simulink model "Modelo_SS_Simulink"  (R2025b)
settings: Solver=ode45  StartTime=0.0  StopTime=inf  FixedStep=0.002  RelTol=1e-3
values from neighbouring files (symbols this model uses):
  A = sym(zeros(7,7))    [Analisis_Contr_Obs.m]    (also in Gs_simbolica.m; Modelo_SS.m = zeros(7,7))
  B_SS = [Bc Bd]    [Modelo_SS.m]
  Bc = sym(zeros(7,1))    [Analisis_Contr_Obs.m]    (also in Modelo_SS.m = zeros(7,1))
  C_s = [0 0 0 1 0 0 0]    [Modelo_SS.m]
  C_SS = eye(7)    [Modelo_SS.m]
  D_SS = zeros(7,4)    [Modelo_SS.m]
  Ff_cte = 9    [Modelo_SS.m]
  K_lqr = lqr(A, Bc, Qx, Qu)    [Modelo_SS.m]
  Kf = 26000    [Modelo_SS.m]
  kr = -1 / (C_p * ((A - Bc*K_lqr) \ Bc))    [Modelo_SS.m]
  Kt = 0.6    [Modelo_SS.m]
  rL = 0.115    [Modelo_SS.m]
  Rm = 0.135    [Modelo_SS.m]
  rP = rP_kin    (= 0.00509295817894)    [Modelo_SS.m]
  tau_sensor = 0.001    [Modelo_SS.m]
  Tf_cte = 2    [Modelo_SS.m]
  Ts_sensor = 0.01    [Modelo_SS.m]
  Vm_max = 48    [Modelo_SS.m]
undefined symbols (not defined in the file or in its folder): L
libraries: simulink_extras x7, sl3dlib x3, dspnetwork x2, simulink x1, hostiolib x1
settings Model: Creator=rodri  LastModifiedBy=rodri
settings RTWCC: GPUComputeCapability=3.5

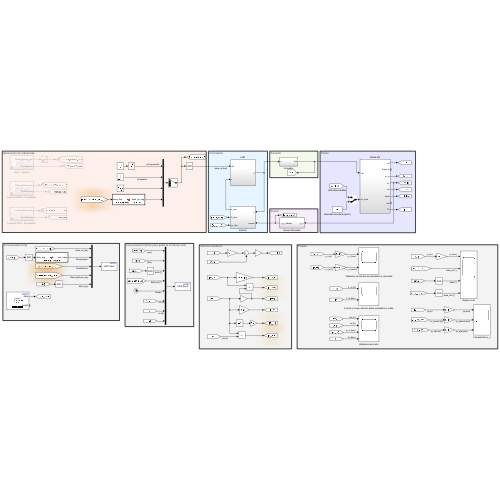
[thumbnail: Simulink's stored preview of the top-level diagram]
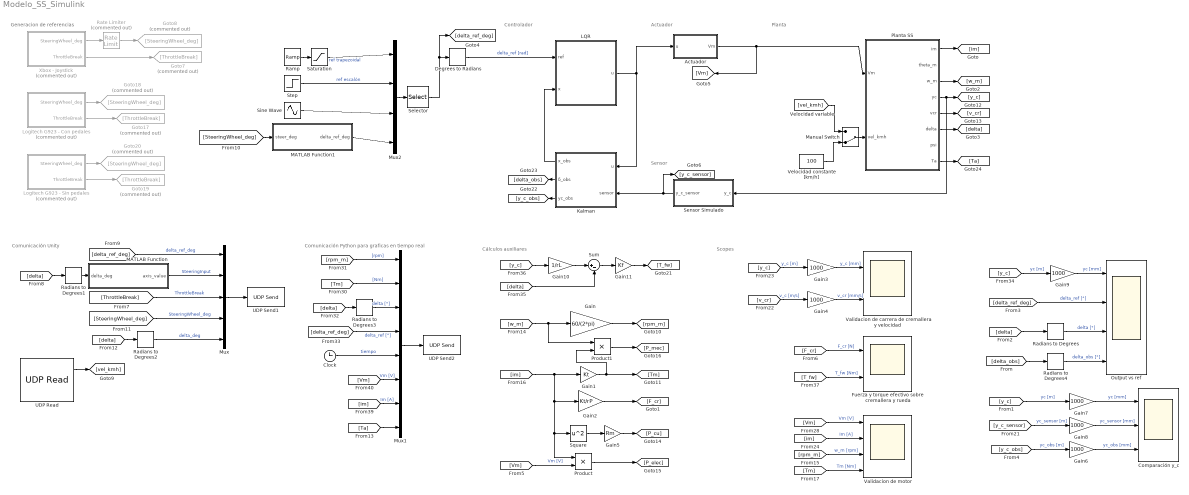
== system Modelo_SS_Simulink ==
  note: Cálculos auxiliares
  note: Scopes
  note: Generacion de referencias
  note: Sensor
  note: Actuador
  note: Comunicación Python para graficas en tiempo real
  note: Comunicación Unity
  note: Controlador
  note: Planta
  Actuador : Subsystem
  Clock : Clock
  Comparación y_c : Scope  NumInputPorts=3
      settings: ActiveDisplayYMinimum=-8.8687499999999986  ActiveDisplayYMaximum=79.158750000000012
  Degrees to Radians : simulink_extras/Transformations/Degrees to Radians
  Fuerza y torque efectivo sobre cremallera y rueda : Scope  NumInputPorts=2
      settings: ActiveDisplayYMinimum=-628.035206695455  ActiveDisplayYMaximum=5652.3168602590958  DataLoggingVariableName=ScopeData7
  Gain : Gain  Gain=60/(2*pi)
  Gain1 : Gain  Gain=Kt
  Gain10 : Gain  Gain=1/rL
  Gain11 : Gain  Gain=Kf
  Gain2 : Gain  Gain=Kt/rP
  Gain{3..4,6..9} (6 alike) : Gain  Gain=1000
  Gain5 : Gain  Gain=Rm
  Goto17 : Goto  Commented=on  GotoTag=ThrottleBreak
  Goto18 : Goto  Commented=on  GotoTag=SteeringWheel_deg
  Goto19 : Goto  Commented=on  GotoTag=ThrottleBreak
  Goto20 : Goto  Commented=on  GotoTag=SteeringWheel_deg
  Goto7 : Goto  Commented=on  GotoTag=ThrottleBreak
  Goto8 : Goto  Commented=on  GotoTag=SteeringWheel_deg
  Kalman : Subsystem
  LQR : Subsystem
  Logitech G923 - Con pedales : Subsystem  Commented=on
  Logitech G923 - Sin pedales : Subsystem  Commented=on
  MATLAB Function : MATLAB Function  TreatAsAtomicUnit=on
  MATLAB Function1 : MATLAB Function  TreatAsAtomicUnit=on
  Manual Switch : ManualSwitch  CurrentSetting=0
  Mux : Mux  Inputs=5
  Mux1 : Mux  Inputs=8
  Mux2 : Mux
  Output vs ref : Scope  NumInputPorts=4
      settings: ActiveDisplayYMinimum=32.897215927252759  ActiveDisplayYMaximum=35.8564863633877
  Planta SS : Subsystem
  Product : Product
  Product1 : Product
  Radians to Degrees{,1..4} (5 alike) : simulink_extras/Transformations/Radians to Degrees
  Ramp : simulink/Sources/Ramp  slope=2000  start=0  InitialOutput=0
  Rate Limiter : RateLimiter  Commented=on  RisingSlewLimit=800  FallingSlewLimit=-800  SampleTimeMode=inherited
  Saturation : Saturate  UpperLimit=35  LowerLimit=-35
  Selector : Selector  InputPortWidth=4  IndexOptions=Index vector (dialog)  Indices=1  OutputSizes=1
  Sensor Simulado : Subsystem
  Sine Wave : Sin  Amplitude=35  Frequency=4.9906  SampleTime=0
  Square : Math  Operator=square
  Step : Step  Time=0  After=35  SampleTime=0
  Sum : Sum  Inputs=|+-
  UDP Read : hostiolib/UDP Read  localURL='0.0.0.0'  localPort=5006  remoteURL='127.0.0.1'  remotePort=-1  recvBufferSize=8192  dims=1  signalDatatype=double  isVarSize=off  showBlockingTime=on  blockingTime=0  sampletime=0.02  blockPlatform=HOST  hoistedMaskSrc=UDP Read/UDP Read Sim/UDP Read
  UDP Send1 : dspnetwork/UDP Send  remoteURL='127.0.0.1'  remotePort=5005  localURL='0.0.0.0'  localPortSource=Automatically determine  localPort=-1  sendBufferSize=8192  sampletime=-1  blockPlatform=HOST  separateLengthPort=0
  UDP Send2 : dspnetwork/UDP Send  remoteURL='172.18.132.160'  remotePort=5010  localURL='0.0.0.0'  localPortSource=Automatically determine  localPort=-1  sendBufferSize=8192  sampletime=-1  blockPlatform=HOST  separateLengthPort=0
  Validacion de carrera de cremallera y velocidad : Scope  NumInputPorts=2
      settings: ActiveDisplayYMinimum=-23.178104837160731  ActiveDisplayYMaximum=208.60294353444661  DataLoggingVariableName=ScopeData5
  Validacion de motor : Scope  NumInputPorts=4
      settings: ActiveDisplayYMinimum=-5.3309284043371674  ActiveDisplayYMaximum=47.978355639034518  DataLoggingVariableName=ScopeData2
  Velocidad constante [km/h] : Constant  Value=100
  Xbox - Joystick : Subsystem  Commented=on
  wires:
  Sine Wave/1 -> Mux2/3
  Radians to Degrees/1 -> Output vs ref/3  "delta [°]"
  Degrees to Radians/1 -> LQR/1(ref)  "delta_ref [rad]"
  Actuador/1(Vm) -> Planta SS/1(Vm), [Vm]
  Sensor Simulado/1("  y_c_sensor") -> Kalman/2(sensor), [y_c_sensor]
  Kalman/1(x_obs) -> LQR/2(x)
  Planta SS/1(im) -> [im]
  [delta] -> Radians to Degrees/1
  [delta_ref_deg] -> Output vs ref/2  "delta_ref [°]"
  Planta SS/3(w_m) -> [w_m]
  Planta SS/6(delta) -> [delta]
  Mux/1 -> UDP Send1/1
  Xbox - Joystick/2(ThrottleBreak) -> Goto7/1
  [ThrottleBreak] -> Mux/3  "ThrottleBreak"
  [delta] -> Radians to Degrees1/1
  MATLAB Function/1(axis_value) -> Mux/2  "SteeringInput"
  [delta_ref_deg] -> Mux/1  "delta_ref_deg"
  Radians to Degrees1/1 -> MATLAB Function/1(delta_deg)
  Xbox - Joystick/1(SteeringWheel_deg) -> Rate Limiter/1
  [SteeringWheel_deg] -> MATLAB Function1/1(steer_deg)
  MATLAB Function1/1(delta_ref_deg) -> Mux2/4
  [SteeringWheel_deg] -> Mux/4  "SteeringWheel_deg"
  [delta] -> Radians to Degrees2/1
  Radians to Degrees2/1 -> Mux/5  "delta_deg"
  UDP Read/1 -> [vel_kmh]
  Velocidad constante [km/h]/1 -> Manual Switch/2
  Selector/1 -> Degrees to Radians/1, [delta_ref_deg]
  [w_m] -> Product1/1, Gain/1
  Gain/1 -> [rpm_m]
  [rpm_m] -> Validacion de motor/3  "w_m [rpm]"
  [im] -> Product/1, Square/1, Gain2/1, Gain1/1
  Gain1/1 -> Product1/2, [Tm]
  [Tm] -> Validacion de motor/4  "Tm [Nm]"
  [y_c] -> Gain7/1  "yc [m]"
  [y_c_sensor] -> Gain8/1  "yc_sensor [m]"
  Planta SS/4(yc) -> Sensor Simulado/1("  y_c"), [y_c]
  Step/1 -> Mux2/2  "ref escalón"
  LQR/1(u) -> Kalman/1(u), Actuador/1(u)
  Gain2/1 -> [F_cr]
  [F_cr] -> Fuerza y torque efectivo sobre cremallera y rueda/1  "F_cr [N]"
  Planta SS/5(vcr) -> [v_cr]
  [v_cr] -> Gain4/1  "v_c [m/s]"
  [y_c] -> Gain3/1  "y_c [m]"
  Gain3/1 -> Validacion de carrera de cremallera y velocidad/1  "y_c [mm]"
  Gain4/1 -> Validacion de carrera de cremallera y velocidad/2  "v_cr [mm/s]"
  [im] -> Validacion de motor/2  "Im [A]"
  Square/1 -> Gain5/1
  Gain5/1 -> [P_cu]
  [Vm] -> Product/2  "Vm [V]"
  Product/1 -> [P_elec]
  Product1/1 -> [P_mec]
  [Vm] -> Validacion de motor/1  "Vm [V]"
  Ramp/1 -> Saturation/1
  Saturation/1 -> Mux2/1  "ref trapezoidal"
  Mux1/1 -> UDP Send2/1
  [rpm_m] -> Mux1/1  "[rpm]"
  [Tm] -> Mux1/2  "[Nm]"
  Logitech G923 - Con pedales/1(SteeringWheel_deg) -> Goto18/1
  Logitech G923 - Con pedales/2(ThrottleBreak) -> Goto17/1
  [delta] -> Radians to Degrees3/1
  Radians to Degrees3/1 -> Mux1/3  "delta [°]"
  [delta_ref_deg] -> Mux1/4  "delta_ref [°]"
  Clock/1 -> Mux1/5  "tiempo"
  Logitech G923 - Sin pedales/2(ThrottleBreak) -> Goto19/1
  Logitech G923 - Sin pedales/1(SteeringWheel_deg) -> Goto20/1
  Gain7/1 -> Comparación y_c/1  "yc [mm]"
  Gain8/1 -> Comparación y_c/2  "yc_sensor [mm]"
  Gain9/1 -> Output vs ref/1  "yc [mm]"
  [y_c] -> Gain9/1  "yc [m]"
  [y_c] -> Gain10/1
  Gain10/1 -> Sum/1
  [delta] -> Sum/2
  Sum/1 -> Gain11/1
  Gain11/1 -> [T_fw]
  [T_fw] -> Fuerza y torque efectivo sobre cremallera y rueda/2  "T_fw [Nm]"
  Rate Limiter/1 -> Goto8/1
  [Vm] -> Mux1/6  "Vm [V]"
  [im] -> Mux1/7  "Im [A]"
  Mux2/1 -> Selector/1
  Manual Switch/1 -> Planta SS/2(vel_kmh)
  [vel_kmh] -> Manual Switch/1
  Kalman/3(yc_obs) -> [y_c_obs]
  Kalman/2(δ_obs) -> [delta_obs]
  [y_c_obs] -> Gain6/1  "yc_obs [m]"
  Gain6/1 -> Comparación y_c/3  "yc_obs [mm]"
  [delta_obs] -> Radians to Degrees4/1
  Radians to Degrees4/1 -> Output vs ref/4  "delta_obs [°]"
  Planta SS/8(Ta) -> [Ta]
  [Ta] -> Mux1/8

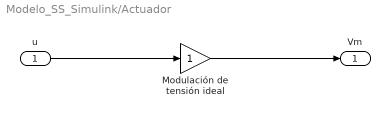
== system Modelo_SS_Simulink/Actuador ==
  u : Inport
  Modulación de tensión ideal : Gain
  Vm : Outport
  wires:
  u/1 -> Modulación de tensión ideal/1
  Modulación de tensión ideal/1 -> Vm/1

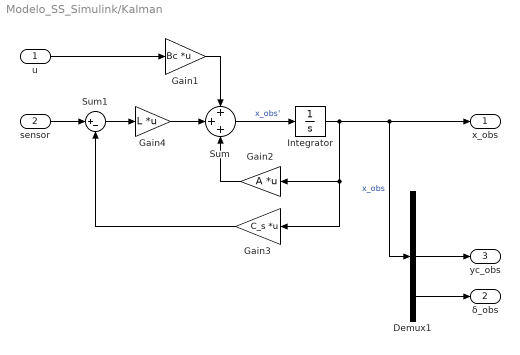
== system Modelo_SS_Simulink/Kalman ==
  u : Inport
  sensor : Inport  Port=2
  Demux1 : Demux  Outputs=7
  Gain1 : Gain  Gain=Bc  Multiplication=Matrix(K*u)
  Gain2 : Gain  Gain=A  Multiplication=Matrix(K*u)
  Gain3 : Gain  Gain=C_s  Multiplication=Matrix(K*u)
  Gain4 : Gain  Gain=L  Multiplication=Matrix(K*u)
  Integrator : Integrator
  Sum : Sum  Inputs=+++
  Sum1 : Sum  Inputs=|+-
  x_obs : Outport
  δ_obs : Outport  Port=2
  yc_obs : Outport  Port=3
  wires:
  Gain1/1 -> Sum/1
  Gain4/1 -> Sum/2
  Sum1/1 -> Gain4/1
  Gain2/1 -> Sum/3
  Integrator/1 -> Gain3/1, Gain2/1, x_obs/1, Demux1/1  "x_obs"
  Gain3/1 -> Sum1/2
  Sum/1 -> Integrator/1  "x_obs'"
  sensor/1 -> Sum1/1
  Demux1/6 -> δ_obs/1
  Demux1/4 -> yc_obs/1
  u/1 -> Gain1/1

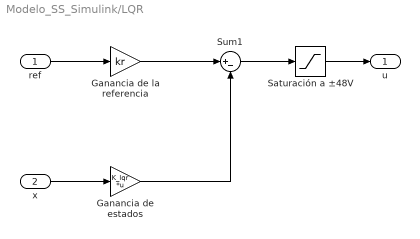
== system Modelo_SS_Simulink/LQR ==
  ref : Inport
  x : Inport  Port=2  PortDimensions=[7]
  Ganancia de estados : Gain  Gain=K_lqr  Multiplication=Matrix(K*u)
  Ganancia de la referencia : Gain  Gain=kr
  Saturación a ±48V : Saturate  UpperLimit=Vm_max  LowerLimit=-Vm_max
  Sum1 : Sum  Inputs=|+-
  u : Outport
  wires:
  ref/1 -> Ganancia de la referencia/1
  Sum1/1 -> Saturación a ±48V/1
  Ganancia de estados/1 -> Sum1/2
  x/1 -> Ganancia de estados/1
  Ganancia de la referencia/1 -> Sum1/1
  Saturación a ±48V/1 -> u/1

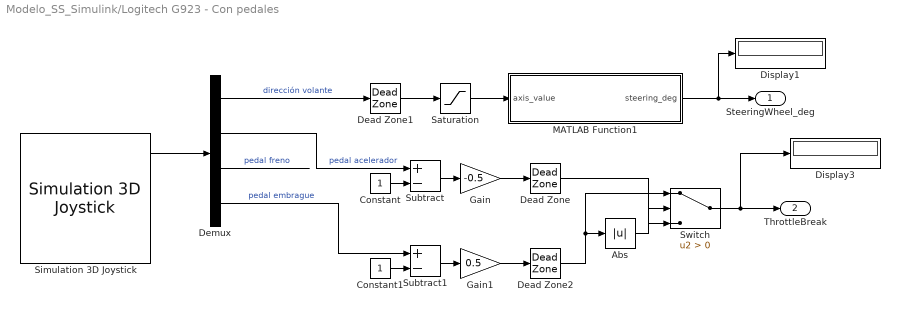
== system Modelo_SS_Simulink/Logitech G923 - Con pedales ==
  Abs : Abs  SaturateOnIntegerOverflow=off
  Constant : Constant
  Constant1 : Constant
  Dead Zone : DeadZone  LowerValue=-1  UpperValue=0.01
  Dead Zone1 : DeadZone  LowerValue=-0.001  UpperValue=0.001
  Dead Zone2 : DeadZone  LowerValue=-0.01  UpperValue=1
  Demux : Demux
  Display1 : Display
  Display3 : Display
  Gain : Gain  Gain=-0.5
  Gain1 : Gain  Gain=0.5
  MATLAB Function1 : MATLAB Function  TreatAsAtomicUnit=on
  Saturation : Saturate  UpperLimit=0.4  LowerLimit=-0.4
  Simulation 3D Joystick : sl3dlib/Simulation 3D/Hardware Interface/Simulation 3D Joystick  joyid=1  adjustports=on  forcefeed=off
  Subtract : Sum  Inputs=+-
  Subtract1 : Sum  Inputs=+-
  Switch : Switch  Criteria=u2 > Threshold  SaturateOnIntegerOverflow=off  InputSameDT=off
  SteeringWheel_deg : Outport
  ThrottleBreak : Outport  Port=2
  wires:
  Demux/1 -> Dead Zone1/1  "dirección volante"
  Simulation 3D Joystick/1 -> Demux/1
  Gain/1 -> Dead Zone/1
  Demux/2 -> Subtract/1  "pedal acelerador"
  Dead Zone1/1 -> Saturation/1
  MATLAB Function1/1(steering_deg) -> Display1/1, SteeringWheel_deg/1
  Saturation/1 -> MATLAB Function1/1(axis_value)
  Constant/1 -> Subtract/2
  Subtract/1 -> Gain/1
  Dead Zone/1 -> Switch/3
  Demux/4 -> Subtract1/1  "pedal embrague"
  Demux/3 -> ?  "pedal freno"
  Constant1/1 -> Subtract1/2
  Dead Zone2/1 -> Switch/1, Abs/1
  Subtract1/1 -> Gain1/1
  Gain1/1 -> Dead Zone2/1
  Abs/1 -> Switch/2
  Switch/1 -> Display3/1, ThrottleBreak/1

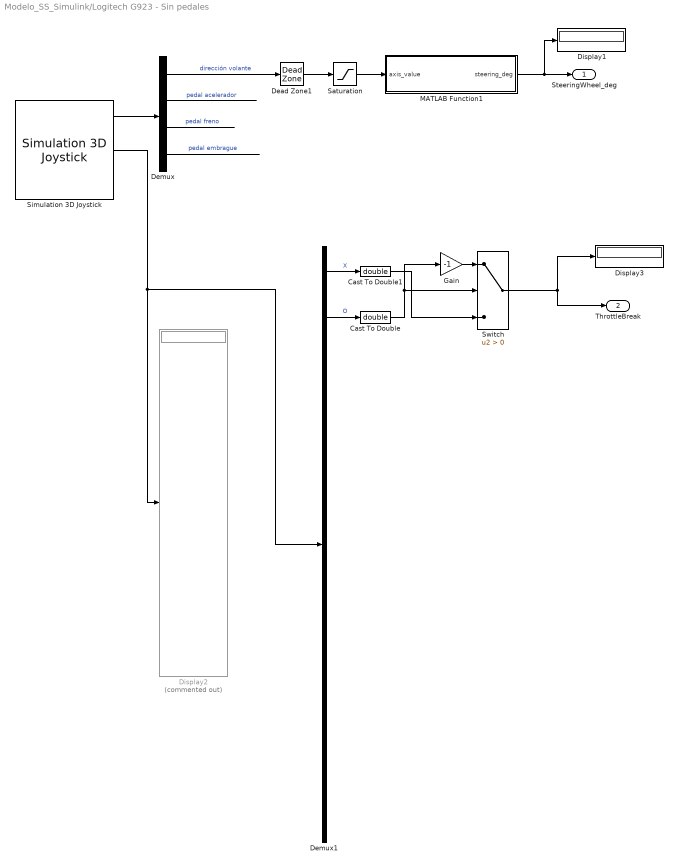
== system Modelo_SS_Simulink/Logitech G923 - Sin pedales ==
  Cast To Double : DataTypeConversion  OutDataTypeStr=double  SaturateOnIntegerOverflow=off  RndMeth=Floor
  Cast To Double1 : DataTypeConversion  OutDataTypeStr=double  SaturateOnIntegerOverflow=off  RndMeth=Floor
  Dead Zone1 : DeadZone  LowerValue=-0.001  UpperValue=0.001
  Demux : Demux
  Demux1 : Demux  Outputs=25
  Display1 : Display
  Display2 : Display  Commented=on
  Display3 : Display
  Gain : Gain  Gain=-1
  MATLAB Function1 : MATLAB Function  TreatAsAtomicUnit=on
  Saturation : Saturate  UpperLimit=0.4  LowerLimit=-0.4
  Simulation 3D Joystick : sl3dlib/Simulation 3D/Hardware Interface/Simulation 3D Joystick  joyid=1  adjustports=on  forcefeed=off
  Switch : Switch  Criteria=u2 > Threshold  SaturateOnIntegerOverflow=off  InputSameDT=off
  SteeringWheel_deg : Outport
  ThrottleBreak : Outport  Port=2
  wires:
  Demux/1 -> Dead Zone1/1  "dirección volante"
  Simulation 3D Joystick/1 -> Demux/1
  Demux/2 -> ?  "pedal acelerador"
  Dead Zone1/1 -> Saturation/1
  MATLAB Function1/1(steering_deg) -> Display1/1, SteeringWheel_deg/1
  Saturation/1 -> MATLAB Function1/1(axis_value)
  Demux/4 -> ?  "pedal embrague"
  Demux/3 -> ?  "pedal freno"
  Simulation 3D Joystick/2 -> Demux1/1, Display2/1
  Demux1/1 -> Cast To Double1/1  "X"
  Switch/1 -> ThrottleBreak/1, Display3/1
  Demux1/3 -> Cast To Double/1  "O"
  Cast To Double/1 -> Gain/1, Switch/2
  Cast To Double1/1 -> Switch/3
  Gain/1 -> Switch/1

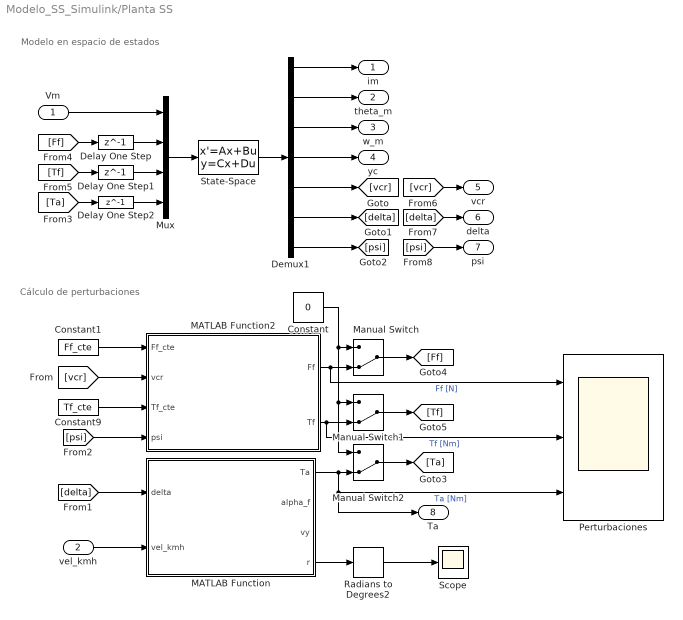
== system Modelo_SS_Simulink/Planta SS ==
  note: Modelo en espacio de estados
  note: Cálculo de perturbaciones
  Vm : Inport
  vel_kmh : Inport  Port=2
  Constant : Constant  Value=0
  Constant1 : Constant  Value=Ff_cte
  Constant9 : Constant  Value=Tf_cte
  Delay One Step : Delay  DelayLength=1
  Delay One Step1 : Delay  DelayLength=1
  Delay One Step2 : Delay  DelayLength=1
  Demux1 : Demux  Outputs=7
  MATLAB Function : MATLAB Function  TreatAsAtomicUnit=on
  MATLAB Function2 : MATLAB Function  TreatAsAtomicUnit=on
  Manual Switch : ManualSwitch  CurrentSetting=0
  Manual Switch1 : ManualSwitch  CurrentSetting=0
  Manual Switch2 : ManualSwitch  CurrentSetting=0
  Mux : Mux
  Perturbaciones : Scope  NumInputPorts=3
      settings: ActiveDisplayString=3  ActiveDisplayYMinimum=-8.942208360008836  ActiveDisplayYMaximum=80.479875240079537
  Radians to Degrees2 : simulink_extras/Transformations/Radians to Degrees
  Scope : Scope
      settings: ActiveDisplayYMinimum=-16.65598559255147  ActiveDisplayYMaximum=149.83624641219754
  State-Space : StateSpace  A=A  B=B_SS  C=C_SS  D=D_SS  InitialCondition=0
  im : Outport
  theta_m : Outport  Port=2
  w_m : Outport  Port=3
  yc : Outport  Port=4
  vcr : Outport  Port=5
  delta : Outport  Port=6
  psi : Outport  Port=7
  Ta : Outport  Port=8
  wires:
  Constant1/1 -> MATLAB Function2/1(Ff_cte)
  State-Space/1 -> Demux1/1
  Constant9/1 -> MATLAB Function2/3(Tf_cte)
  Mux/1 -> State-Space/1
  Vm/1 -> Mux/1
  Demux1/1 -> im/1
  Demux1/2 -> theta_m/1
  Demux1/3 -> w_m/1
  Demux1/4 -> yc/1
  [vcr] -> MATLAB Function2/2(vcr)
  Demux1/5 -> [vcr]
  Demux1/6 -> [delta]
  [delta] -> MATLAB Function/1(delta)
  Demux1/7 -> [psi]
  [psi] -> MATLAB Function2/4(psi)
  [Ta] -> Delay One Step2/1
  MATLAB Function2/1(Ff) -> Perturbaciones/1, Manual Switch/2  "Ff [N]"
  MATLAB Function2/2(Tf) -> Perturbaciones/2, Manual Switch1/2  "Tf [Nm]"
  [Ff] -> Delay One Step/1
  [Tf] -> Delay One Step1/1
  [vcr] -> vcr/1
  [delta] -> delta/1
  [psi] -> psi/1
  Manual Switch/1 -> [Ff]
  Manual Switch2/1 -> [Ta]
  Manual Switch1/1 -> [Tf]
  Constant/1 -> Manual Switch2/1, Manual Switch1/1, Manual Switch/1
  Delay One Step/1 -> Mux/2
  Delay One Step1/1 -> Mux/3
  Delay One Step2/1 -> Mux/4
  Radians to Degrees2/1 -> Scope/1
  vel_kmh/1 -> MATLAB Function/2(vel_kmh)
  MATLAB Function/1(Ta) -> Ta/1, Perturbaciones/3, Manual Switch2/2  "Ta [Nm]"
  MATLAB Function/4(r) -> Radians to Degrees2/1

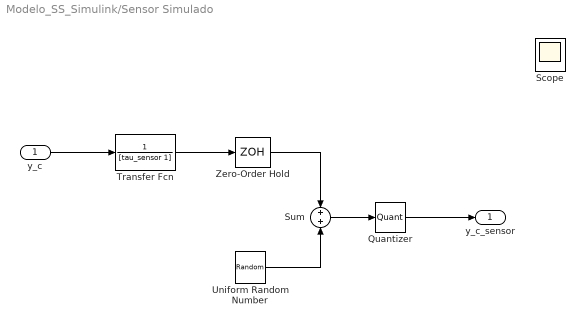
== system Modelo_SS_Simulink/Sensor Simulado ==
  "  y_c" : Inport
  " Quantizer" : Quantizer  QuantizationInterval=q_yc
  " Transfer Fcn" : TransferFcn  Denominator=[tau_sensor 1]
  " Uniform Random Number" : UniformRandomNumber  Minimum=-0.135e-3  Maximum=0.135e-3  SampleTime=Ts_sensor
  " Zero-Order Hold" : ZeroOrderHold  SampleTime=Ts_sensor
  Scope : Scope  NumInputPorts=2
      settings: ActiveDisplayYMinimum=-0.0088687499999999982  ActiveDisplayYMaximum=0.07915875  DataLoggingVariableName=ScopeData4
  Sum : Sum
  "  y_c_sensor" : Outport
  wires:
  " Transfer Fcn"/1 -> " Zero-Order Hold"/1
  "  y_c"/1 -> " Transfer Fcn"/1
  " Zero-Order Hold"/1 -> Sum/1
  Sum/1 -> " Quantizer"/1
  " Quantizer"/1 -> "  y_c_sensor"/1
  " Uniform Random Number"/1 -> Sum/2

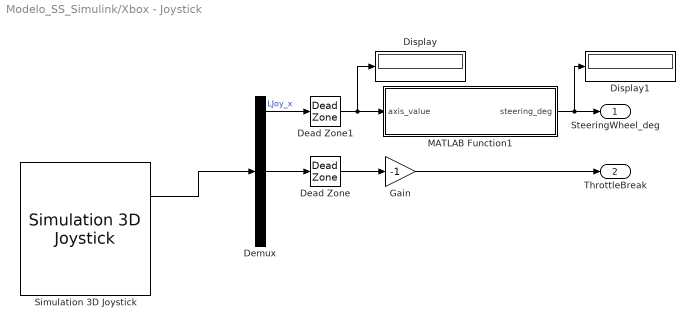
== system Modelo_SS_Simulink/Xbox - Joystick ==
  Dead Zone : DeadZone  LowerValue=-0.1  UpperValue=0.1
  Dead Zone1 : DeadZone  LowerValue=-0.1  UpperValue=0.1
  Demux : Demux  Outputs=5
  Display : Display
  Display1 : Display
  Gain : Gain  Gain=-1
  MATLAB Function1 : MATLAB Function  TreatAsAtomicUnit=on
  Simulation 3D Joystick : sl3dlib/Simulation 3D/Hardware Interface/Simulation 3D Joystick  joyid=1  adjustports=on  forcefeed=off
  SteeringWheel_deg : Outport
  ThrottleBreak : Outport  Port=2
  wires:
  Demux/1 -> Dead Zone1/1  "LJoy_x"
  Simulation 3D Joystick/1 -> Demux/1
  Demux/3 -> Dead Zone/1
  Gain/1 -> ThrottleBreak/1
  Dead Zone/1 -> Gain/1
  Dead Zone1/1 -> Display/1, MATLAB Function1/1(axis_value)
  MATLAB Function1/1(steering_deg) -> Display1/1, SteeringWheel_deg/1

== matlab function Modelo_SS_Simulink/Logitech G923 - Con pedales/MATLAB Function1 ==
  data: axis_value input; steering_deg output
function steering_deg = gamepad2steeringwheel(axis_value)
% Convierte un valor de gamepad en [-0.4, 0.4]
% a ángulo de volante en grados [-180, 180]
%
% Entrada:
%   axis_value   : valor del eje del gamepad
%
% Salida:
%   steering_deg : ángulo de volante en grados

    steering_max = 180;   % [deg]
    axis_max     = 0.4;

    % Escalado lineal
    steering_deg = (axis_value / axis_max) * steering_max;

end

== matlab function Modelo_SS_Simulink/MATLAB Function1 ==
  data: steer_deg input; delta_ref_deg output
function delta_ref_deg = steeringWheel2deltaRef(steer_deg)
% steeringWheel2deltaRef
% Convierte ángulo de volante [-180,180] [deg]
% a delta_ref [-35,35] [deg]
% usando una ganancia K externa (0 ≤ K ≤ 1 típicamente).
%
% Entradas:
%   steer_deg : ángulo de volante [deg]
%   K         : factor de sensibilidad (ajustado externamente)
%
% Salida:
%   delta_ref_deg : referencia de ángulo de rueda [deg]
    K = 1;

    steer_max = 180;   % [deg]
    delta_max = 35;    % [deg]

    % Si entran vectores (p.ej. [2]), tomo el primer componente
    steer_deg = steer_deg(1);
    K         = K(1);

    steer_deg = max(min(steer_deg, steer_max), -steer_max);
    K = min(max(K, 0), 1);

    delta_ref_deg = (delta_max * K) * (steer_deg / steer_max);
    delta_ref_deg = max(min(delta_ref_deg, delta_max), -delta_max);

end

== matlab function Modelo_SS_Simulink/Planta SS/MATLAB Function2 ==
  data: Ff_cte input; vcr input; Tf_cte input; Ff output; psi input; Tf output
function [Ff, Tf] = PerturbacionesFriccion(Ff_cte, vcr, Tf_cte, psi)

%Ff = sign(vcr) * Ff_cte;
%Tf = sign(psi) * Tf_cte;

v_eps_cr = 1e-1;   % [m/s]
w_eps_f  = 1e-4;   % [rad/s]

Ff = Ff_cte * (2/pi) * atan(vcr / v_eps_cr);
Tf = Tf_cte * (2/pi) * atan(psi / w_eps_f);

== matlab function Modelo_SS_Simulink/MATLAB Function ==
  data: delta_deg input; axis_value output
function axis_value = delta2gamepad(delta_deg)
% Convierte un ángulo delta en grados [-35, 35]
% a un valor normalizado de gamepad [-1, 1]
%
% Entrada:
%   delta_deg  : ángulo en grados
%
% Salida:
%   axis_value : valor normalizado [-1, 1]

    delta_max = 35;  % [deg]

    % Saturación defensiva
    delta_deg = max(min(delta_deg, delta_max), -delta_max);

    % Escalado lineal
    axis_value = delta_deg / delta_max;

end

== matlab function Modelo_SS_Simulink/Xbox - Joystick/MATLAB Function1 ==
  data: axis_value input; steering_deg output
function steering_deg = gamepad2steeringwheel(axis_value)
% Convierte un valor de gamepad en [-1, 1]
% a ángulo de volante en grados [-180, 180]
%
% Entrada:
%   axis_value   : valor normalizado del eje
%
% Salida:
%   steering_deg : ángulo de volante en grados

    steering_max = 180;  % [deg]

    % Saturación defensiva
    axis_value = max(min(axis_value, 1), -1);

    % Escalado lineal
    steering_deg = steering_max * axis_value;

end

== matlab function Modelo_SS_Simulink/Planta SS/MATLAB Function ==
  data: delta input; Ta output; vel_kmh input; alpha_f output; vy output; r output
function [Ta, alpha_f, vy, r] = CalculoTaPorRueda(delta, vel_kmh)
% CalculoTaPorRueda
% Calcula el torque autoalineante por rueda delantera,
% suponiendo que ambas ruedas delanteras tienen el mismo
% angulo y comportamiento.
%
% Entradas:
%   delta    [rad]   angulo de rueda delantera
%   vel_kmh  [km/h]  velocidad vehicular
%
% Salidas:
%   Ta       [N*m]   torque autoalineante por rueda
%   alpha_f  [rad]   slip angle delantero
%   vy       [m/s]   velocidad lateral CG (steady-state)
%   r        [rad/s] yaw rate (steady-state)

    % Parametros vehiculo
    m = 1400;
    g = 9.80665;
    L = 2.70;
    a = 1.20;
    b = L - a;

    % Rigideces por eje para el modelo bicicleta
    Cf_axle = 8e4;   % [N/rad]
    Cr_axle = 8e4;   % [N/rad]

    % Parametros de saturacion / trail
    mu = 0.90;
    t0 = 0.08;       % [m] mantener igual al modelo actual
    kAlpha = 8.0;
    Vt = 40;         % [m/s]

    Vx = vel_kmh / 3.6;

    if Vx < 0.5
        Ta = 0;
        alpha_f = 0;
        vy = 0;
        r = 0;
        return
    end

    Vx_eff = max(Vx, 0.5);

    % Modelo bicicleta en regimen estacionario
    M11 = Cf_axle + Cr_axle;
    M12 = m * Vx_eff^2 + Cf_axle * a - Cr_axle * b;

    M21 = a * Cf_axle - b * Cr_axle;
    M22 = a^2 * Cf_axle + b^2 * Cr_axle;

    rhs1 = Cf_axle * Vx_eff * delta;
    rhs2 = a * Cf_axle * Vx_eff * delta;

    M = [M11, M12; M21, M22];
    rhs = [rhs1; rhs2];

    sol = M \ rhs;
    vy = sol(1);
    r = sol(2);

    % Slip delantero comun a ambas ruedas
    alpha_f = delta - (vy + a * r) / Vx_eff;

    % Conversion a magnitudes por rueda
    Cf_wheel = Cf_axle / 2;
    Fzf_wheel = ((b / L) * m * g) / 2;
    Fy_max_wheel = mu * Fzf_wheel;

    % Fuerza lateral por rueda con saturacion suave
    Fy_lin_wheel = Cf_wheel * alpha_f;
    Fy_wheel = Fy_max_wheel * tanh(Fy_lin_wheel / Fy_max_wheel);

    % Trail efectivo
    trail = t0 * exp(-kAlpha * abs(alpha_f)) * (1 / (1 + (Vx_eff / Vt)^2));

    % Torque autoalineante por rueda
    Ta = Fy_wheel * trail;
end

== matlab function Modelo_SS_Simulink/Logitech G923 - Sin pedales/MATLAB Function1 ==
  data: axis_value input; steering_deg output
function steering_deg = gamepad2steeringwheel(axis_value)
% Convierte un valor de gamepad en [-0.4, 0.4]
% a ángulo de volante en grados [-180, 180]
%
% Entrada:
%   axis_value   : valor del eje del gamepad
%
% Salida:
%   steering_deg : ángulo de volante en grados

    steering_max = 180;   % [deg]
    axis_max     = 0.4;

    % Escalado lineal
    steering_deg = (axis_value / axis_max) * steering_max;

end
